simulink model "szabalyozo"  (R2021a)
settings: Solver=VariableStepAuto  StartTime=0.0  StopTime=0.5  RelTol=1e-3
values from neighbouring files (symbols this model uses):
  Ad = [-0.6 0 0 ... (first row only)    [folyamar.m]    (also in szamol.m = tetam(1:3,1:3)')
  Bd = [-2 ... (first row only)    [folyamar.m]    (also in szamol.m = tetam(4,:)')
  Cd = [1 1 -1]    [folyamar.m]    (also in szamol.m)
  teta = teta+K*e    [becslo.m]    (also in folyamar.m = [Ad' ; Bd'])
settings Model: Creator=Krisz  LastModifiedBy=Krisz

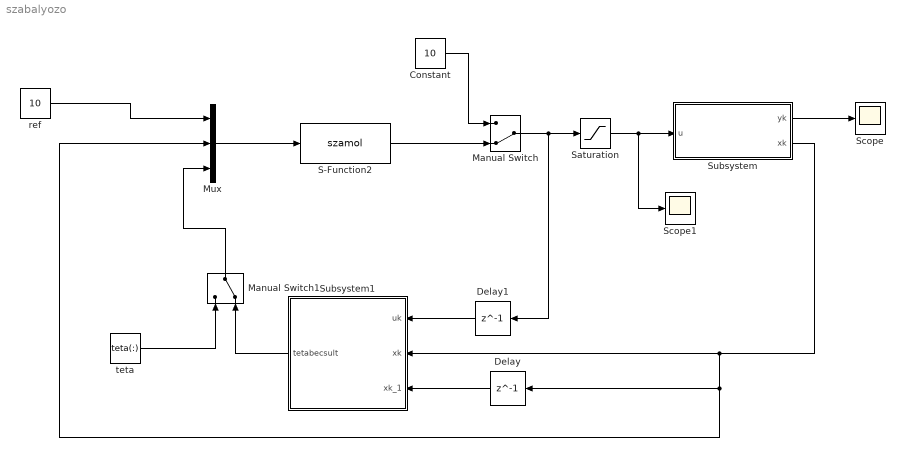
== system szabalyozo ==
  Constant : Constant  Value=10
  Delay : Delay  DelayLength=1  InitialCondition=0
  Delay1 : Delay  DelayLength=1  InitialCondition=0
  Manual Switch : ManualSwitch  CurrentSetting=0
  Manual Switch1 : ManualSwitch  CurrentSetting=0
  Mux : Mux  Inputs=3
  S-Function2 : S-Function  FunctionName=szamol  SFunctionDeploymentMode=off  EnableBusSupport=off
  Saturation : Saturate  UpperLimit=50  LowerLimit=-50
  Scope : Scope
  Scope1 : Scope
  Subsystem : Subsystem  mask{Ad=Ad, Bd=Bd, Cd=Cd}
  Subsystem1 : Subsystem  mask{Ad=Ad, Bd=Bd, Cd=Cd}
  ref : Constant  Value=10
  teta : Constant  Value=teta(:)
  wires:
  Manual Switch/1 -> Delay1/1, Saturation/1
  Constant/1 -> Manual Switch/1
  Subsystem/1(yk) -> Scope/1
  S-Function2/1 -> Manual Switch/2
  ref/1 -> Mux/1
  Mux/1 -> S-Function2/1
  Subsystem/2(xk) -> Subsystem1/2(xk), Delay/1, Mux/2
  teta/1 -> Manual Switch1/1
  Manual Switch1/1 -> Mux/3
  Subsystem1/1(tetabecsult) -> Manual Switch1/2
  Delay/1 -> Subsystem1/3(xk_1)
  Saturation/1 -> Scope1/1, Subsystem/1(u)
  Delay1/1 -> Subsystem1/1(uk)

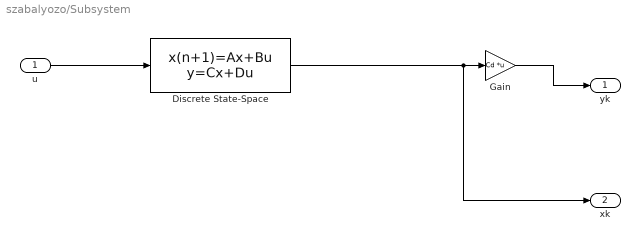
== system szabalyozo/Subsystem ==
  u : Inport
  Discrete State-Space : DiscreteStateSpace  A=Ad  B=Bd  C=eye(3)  D=zeros(3,1)  SampleTime=-1
  Gain : Gain  Gain=Cd  Multiplication=Matrix(K*u)
  yk : Outport
  xk : Outport  Port=2
  wires:
  Discrete State-Space/1 -> Gain/1, xk/1
  u/1 -> Discrete State-Space/1
  Gain/1 -> yk/1

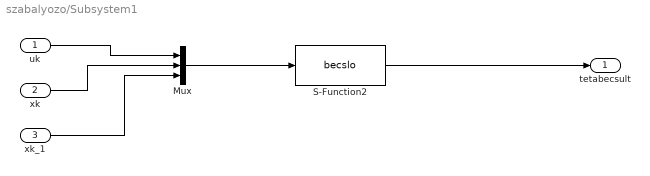
== system szabalyozo/Subsystem1 ==
  uk : Inport
  xk : Inport  Port=2
  xk_1 : Inport  Port=3
  Mux : Mux  Inputs=3
  S-Function2 : S-Function  FunctionName=becslo  SFunctionDeploymentMode=off  EnableBusSupport=off
  tetabecsult : Outport
  wires:
  uk/1 -> Mux/1
  xk/1 -> Mux/2
  Mux/1 -> S-Function2/1
  S-Function2/1 -> tetabecsult/1
  xk_1/1 -> Mux/3
